simulink model "S4_LP_SCR_bypass_2018b"  (R2018b)
settings: Solver=VariableStepAuto  StartTime=0.0  StopTime=20000  RelTol=1e-3
undefined symbols (not defined in the file or in its folder): sigbuilder_block
libraries: fl_lib x70, sh_lib x49, nesl_utility x29
(part 2 of 2)

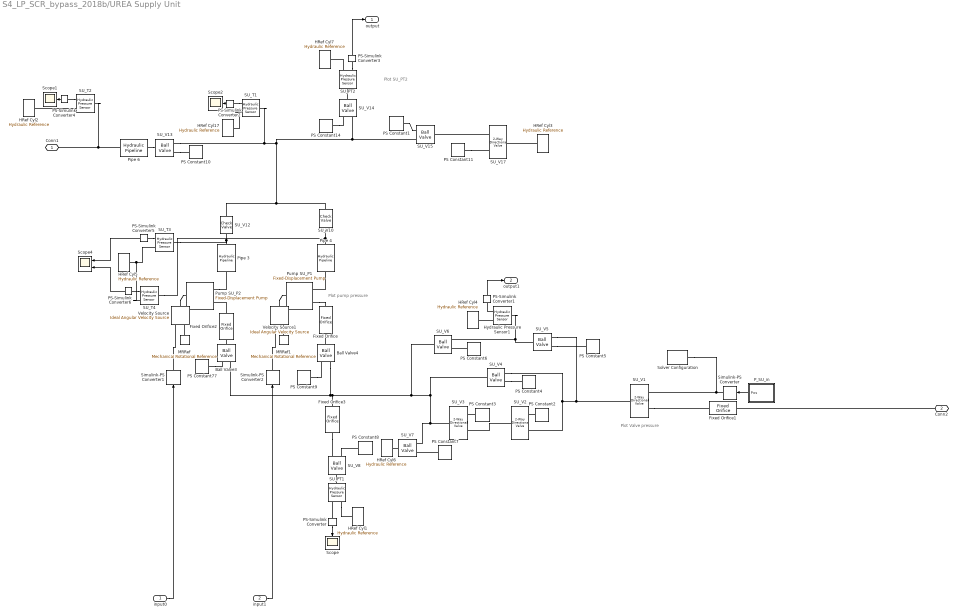
== system S4_LP_SCR_bypass_2018b/UREA Supply Unit ==
  note: Plot Valve pressure
  note: Plot pump pressure
  note: Plot SU_PT2
  input0 : Inport
  input1 : Inport  Port=2
  Ball Valve3 : sh_lib/Valves/Flow Control Valves/Ball Valve  valve_seat_spec=1  cone_ang=120 deg  d_ball=0.01 m  d_orif=5e-3 m  x_0=0 m  C_d=0.65  A_leak=1e-20 m^2  lam_spec=1  B_lam=0.999  Re_cr=10  flow_rate_specify=off  flow_rate_priority=None  flow_rate=1e-3 m^3/s  flow_rate_nominal_specify=off  flow_rate_nominal_unit=m^3/s  flow_rate_nominal_value=1  pressure_drop_specify=off  pressure_drop_priority=None  pressure_drop=0 Pa  pressure_drop_nominal_specify=off  pressure_drop_nominal_unit=Pa  pressure_drop_nominal_value=1
      settings: SourceProductBaseCode=SH  InternalSimscapePortConfiguration="{\"Bottom\":[],\"Left\":[{\"id\":\"S\",\"label\":\"S\",\"type\":\"input\"},{\"id\":\"A\",\"label\":\"A\",\"type\":\"foundation.hydraulic.hydraulic\"}],\"Right\":[{\"id\":\"B\",\"label\":\"B\",\"type\":\"foundation.hydraulic.hydraulic\"}],\"Top\":[]}"
  Ball Valve4 : sh_lib/Valves/Flow Control Valves/Ball Valve  valve_seat_spec=1  cone_ang=120 deg  d_ball=0.01 m  d_orif=5e-3 m  x_0=0 m  C_d=0.65  A_leak=1e-20 m^2  lam_spec=1  B_lam=0.999  Re_cr=10  flow_rate_specify=off  flow_rate_priority=None  flow_rate=1e-3 m^3/s  flow_rate_nominal_specify=off  flow_rate_nominal_unit=m^3/s  flow_rate_nominal_value=1  pressure_drop_specify=off  pressure_drop_priority=None  pressure_drop=0 Pa  pressure_drop_nominal_specify=off  pressure_drop_nominal_unit=Pa  pressure_drop_nominal_value=1
      settings: SourceProductBaseCode=SH  InternalSimscapePortConfiguration="{\"Bottom\":[],\"Left\":[{\"id\":\"S\",\"label\":\"S\",\"type\":\"input\"},{\"id\":\"A\",\"label\":\"A\",\"type\":\"foundation.hydraulic.hydraulic\"}],\"Right\":[{\"id\":\"B\",\"label\":\"B\",\"type\":\"foundation.hydraulic.hydraulic\"}],\"Top\":[]}"
  Fixed Orifice{,1..3} (4 alike) : sh_lib/Orifices/Fixed Orifice  area=1e-4 m^2  C_d=0.7  lam_spec=1  B_lam=0.999  Re_cr=12  q_specify=off  q_priority=None  q=1e-3 m^3/s  q_nominal_specify=off  q_nominal_unit=m^3/s  q_nominal_value=1  p_specify=off  p_priority=None  p=0 Pa  p_nominal_specify=off  p_nominal_unit=Pa  p_nominal_value=1
      settings: SourceProductBaseCode=SH  InternalSimscapePortConfiguration="{\"Bottom\":[],\"Left\":[{\"id\":\"A\",\"label\":\"A\",\"type\":\"foundation.hydraulic.hydraulic\"}],\"Right\":[{\"id\":\"B\",\"label\":\"B\",\"type\":\"foundation.hydraulic.hydraulic\"}],\"Top\":[]}"
  HRef Cyl{1..7,17} (8 alike) : fl_lib/Hydraulic/Hydraulic Elements/Hydraulic Reference  Tag=Factory Generic
      settings: SourceProductBaseCode=PW,SS,VE
  Hydraulic Pressure Sensor1 : fl_lib/Hydraulic/Hydraulic Sensors/Hydraulic Pressure Sensor
      settings: SourceProductBaseCode=PW,SS,VE
  MRRef : fl_lib/Mechanical/Rotational Elements/Mechanical Rotational Reference  Tag=Factory Generic
      settings: SourceProductBaseCode=PW,SS,VE
  MRRef1 : fl_lib/Mechanical/Rotational Elements/Mechanical Rotational Reference  Tag=Factory Generic
      settings: SourceProductBaseCode=PW,SS,VE
  PS Constant{1..3,6,11,14} (6 alike) : fl_lib/Physical Signals/Sources/PS Constant  constant=1
      settings: SourceProductBaseCode=PW,SS,VE
  PS Constant10 : fl_lib/Physical Signals/Sources/PS Constant  constant=1 m
      settings: SourceProductBaseCode=PW,SS,VE
  PS Constant4 : fl_lib/Physical Signals/Sources/PS Constant  constant=0 m
      settings: SourceProductBaseCode=PW,SS,VE
  PS Constant5 : fl_lib/Physical Signals/Sources/PS Constant  constant=1 m
      settings: SourceProductBaseCode=PW,SS,VE
  PS Constant7 : fl_lib/Physical Signals/Sources/PS Constant  constant=0 m
      settings: SourceProductBaseCode=PW,SS,VE
  PS Constant77 : fl_lib/Physical Signals/Sources/PS Constant  constant=0.01 m
      settings: SourceProductBaseCode=PW,SS,VE
  PS Constant8 : fl_lib/Physical Signals/Sources/PS Constant  constant=1 m
      settings: SourceProductBaseCode=PW,SS,VE
  PS Constant9 : fl_lib/Physical Signals/Sources/PS Constant  constant=0.01 m
      settings: SourceProductBaseCode=PW,SS,VE
  PS-Simulink Converter{,1..6} (7 alike) : nesl_utility/PS-Simulink Converter  PhysicalDomain=network_engine_domain  SubClassName=ps_output  LeftPortType=input  RightPortType=output  PseudoPeriodic=off  Frequencies=[]  VectorFormat=inherit  Unit=inherit  AffineConversion=off
      settings: SourceProductBaseCode=SS,PW,VE
  P_SU_in : Subsystem  Tag=STV Subsys  LoadFcn=sigbuilder_block('load');  StartFcn=sigbuilder_block('start');  StopFcn=sigbuilder_block('stop');  ClipboardFcn=sigbuilder_block('clipboard');  mask(Sigbuilder block){tuvar=[0:10]}
      mask help: Sigbuilder GUI
      mask init:
      | if ~strcmp(get_param(bdroot(gcbh),'SimulationStatus'),'stopped') tuvar = sigbuilder_block('maskInit'); end
      settings: CopyFcn=sigbuilder_block('copy');  DeleteFcn=sigbuilder_block('delete');  ModelCloseFcn=sigbuilder_block('modelClose');  PreSaveFcn=sigbuilder_block('preSave');  PauseFcn=sigbuilder_block('pause')  ContinueFcn=sigbuilder_block('continue')  NameChangeFcn=sigbuilder_block('namechange');  OpenFcn=sigbuilder_block('open',[0 0 787.5 524.25 ]);  CloseFcn=sigbuilder_block('close');
      mask Display: plot(0, 0, 100, 100,[2, 2, 32, 32, 2], [68, 8, 8, 68, 68],[32, 2], [38, 38], [32, 19, 2],[53, 60, 44], [32, 17, 17, 2],[16, 16, 31, 31]);txt = getActiveGroup(gcbh);text(2, 100, txt,'verticalAlignment', 'top');
  Pipe 3 : sh_lib/Pipelines/Hydraulic Pipeline  Tag=Factory Generic  cs_type=1  d_in=0.016 m  area=1e-04 m^2  D_h=0.0112 m  s_factor=64  length=5 m  length_ad=1 m  roughness=1.5e-05 m  Re_lam=2e+03  Re_turb=4e+03  wall_type=1  pr_r_coef=2e-10 m/Pa  time_const=0.008 s  k_sh=1.4  initial_pressure=0 Pa
      settings: SourceProductBaseCode=SH  InternalSimscapePortConfiguration="{\"Bottom\":[],\"Left\":[{\"id\":\"A\",\"label\":\"A\",\"type\":\"foundation.hydraulic.hydraulic\"}],\"Right\":[{\"id\":\"B\",\"label\":\"B\",\"type\":\"foundation.hydraulic.hydraulic\"}],\"Top\":[]}"
  Pipe 4 : sh_lib/Pipelines/Hydraulic Pipeline  Tag=Factory Generic  cs_type=1  d_in=0.015 m  area=1e-04 m^2  D_h=0.0112 m  s_factor=64  length=1 m  length_ad=1 m  roughness=1.5e-06 m  Re_lam=2e+03  Re_turb=4e+03  wall_type=1  pr_r_coef=2e-10 m/Pa  time_const=0.008 s  k_sh=1.4  initial_pressure=0 Pa
      settings: SourceProductBaseCode=SH  InternalSimscapePortConfiguration="{\"Bottom\":[],\"Left\":[{\"id\":\"A\",\"label\":\"A\",\"type\":\"foundation.hydraulic.hydraulic\"}],\"Right\":[{\"id\":\"B\",\"label\":\"B\",\"type\":\"foundation.hydraulic.hydraulic\"}],\"Top\":[]}"
  Pipe 6 : sh_lib/Pipelines/Hydraulic Pipeline  Tag=Factory Generic  cs_type=1  d_in=0.016 m  area=1e-04 m^2  D_h=0.0112 m  s_factor=1  length=5 m  length_ad=1 m  roughness=1.5e-05 m  Re_lam=2e+03  Re_turb=4e+03  wall_type=1  pr_r_coef=2e-10 m/Pa  time_const=0.008 s  k_sh=1.4  initial_pressure=0 Pa
      settings: SourceProductBaseCode=SH  LogSimulationData=on  InternalSimscapePortConfiguration="{\"Bottom\":[],\"Left\":[{\"id\":\"A\",\"label\":\"A\",\"type\":\"foundation.hydraulic.hydraulic\"}],\"Right\":[{\"id\":\"B\",\"label\":\"B\",\"type\":\"foundation.hydraulic.hydraulic\"}],\"Top\":[]}"
  Pump SU_P1 : sh_lib/Pumps and Motors/Fixed-Displacement Pump  D=3.2 cm^3/rev  loss_spec=1  w_nominal=200 rad/s  pr_nominal=5e7 Pa  visc_nominal=18 cSt  dens_nominal=1032.38 kg/m^3  efficiency_vol=0.92  no_load_torque=0.05 N*m  torque_pressure_coeff=0.6e-6 N*m/Pa  p_diff_eff_TLU=[100000, 1000000, 2000000] Pa  omega_eff_TLU=[25, 50, 100, 200, 300, 400] rad/s  vol_eff_TLU=[.816, .908, .954, .977, .981, .984; .325, .663, .831, .916, .925, .946; .137, .568, .78, .892, .893, .91]  mech_eff_TLU=[.996, .996, .996, .996, .996, .996; .988, .989, .989, .989, .989, .99; .981, .981, .982, .982, .983, .984]  p_diff_loss_TLU=[100000, 1000000, 2000000] Pa  omega_loss_TLU=[25, 50, 100, 200, 300, 400] rad/s  vol_loss_TLU=[.023, .023, .023, .023, .0285, .032; .0844, .0842, .0845, .084, .1125, .108; .1079, .108, .11, .108, .1605, .18] * 1e-3 m^3/s  mech_loss_TLU=[.002, .002, .002, .002, .002, .002; .0607, .0556, .0556, .0556, .0556, .0505; .1937, .1937, .1833, .1833, .1729, .1626] N*m  pressure_threshold=1e5 Pa  omega_threshold=10 rad/s  quadrant_check=0  pressure_check=0  min_valid_pressure=0 Pa  vol_eff_min=1e-3  vol_eff_max=1  mech_eff_min=1e-3  mech_eff_max=1
      settings: SourceProductBaseCode=SH  LogSimulationData=on  InternalSimscapePortConfiguration="{\"Bottom\":[],\"Left\":[{\"id\":\"S\",\"label\":\"S\",\"type\":\"foundation.mechanical.rotational.rotational\"}],\"Right\":[{\"id\":\"P\",\"label\":\"P\",\"type\":\"foundation.hydraulic.hydraulic\"},{\"id\":\"T\",\"label\":\"T\",\"type\":\"foundation.hydraulic.hydraulic\"}],\"Top\":[]}"
  Pump SU_P2 : sh_lib/Pumps and Motors/Fixed-Displacement Pump  D=3.2 cm^3/rev  loss_spec=1  w_nominal=188 rad/s  pr_nominal=100e5 Pa  visc_nominal=18 cSt  dens_nominal=900 kg/m^3  efficiency_vol=0.92  no_load_torque=0.05 N*m  torque_pressure_coeff=0.6e-6 N*m/Pa  p_diff_eff_TLU=[100000, 1000000, 2000000] Pa  omega_eff_TLU=[25, 50, 100, 200, 300, 400] rad/s  vol_eff_TLU=[.816, .908, .954, .977, .981, .984; .325, .663, .831, .916, .925, .946; .137, .568, .78, .892, .893, .91]  mech_eff_TLU=[.996, .996, .996, .996, .996, .996; .988, .989, .989, .989, .989, .99; .981, .981, .982, .982, .983, .984]  p_diff_loss_TLU=[100000, 1000000, 2000000] Pa  omega_loss_TLU=[25, 50, 100, 200, 300, 400] rad/s  vol_loss_TLU=[.023, .023, .023, .023, .0285, .032; .0844, .0842, .0845, .084, .1125, .108; .1079, .108, .11, .108, .1605, .18] * 1e-3 m^3/s  mech_loss_TLU=[.002, .002, .002, .002, .002, .002; .0607, .0556, .0556, .0556, .0556, .0505; .1937, .1937, .1833, .1833, .1729, .1626] N*m  pressure_threshold=1e5 Pa  omega_threshold=10 rad/s  quadrant_check=0  pressure_check=0  min_valid_pressure=0 Pa  vol_eff_min=1e-3  vol_eff_max=1  mech_eff_min=1e-3  mech_eff_max=1
      settings: SourceProductBaseCode=SH  InternalSimscapePortConfiguration="{\"Bottom\":[],\"Left\":[{\"id\":\"S\",\"label\":\"S\",\"type\":\"foundation.mechanical.rotational.rotational\"}],\"Right\":[{\"id\":\"P\",\"label\":\"P\",\"type\":\"foundation.hydraulic.hydraulic\"},{\"id\":\"T\",\"label\":\"T\",\"type\":\"foundation.hydraulic.hydraulic\"}],\"Top\":[]}"
  SU_PT1 : fl_lib/Hydraulic/Hydraulic Sensors/Hydraulic Pressure Sensor
      settings: SourceProductBaseCode=PW,SS,VE
  SU_PT2 : fl_lib/Hydraulic/Hydraulic Sensors/Hydraulic Pressure Sensor
      settings: SourceProductBaseCode=PW,SS,VE
  SU_T{1..4} (4 alike) : fl_lib/Hydraulic/Hydraulic Sensors/Hydraulic Pressure Sensor
      settings: SourceProductBaseCode=PW,SS,VE
  SU_V{1..3,17} (4 alike) : sh_lib/Valves/Directional Valves/2-Way Directional Valve  Tag=Factory Generic  mdl_type=1  area_max=2.2e-4 m^2  opening_max=0.01 m  opening_tab="[  -0.002 0 0.005 0.015 ] m"  area_tab="[  1e-12 4e-12 1e-05 1.02e-05 ] m^2"  pressure_tab="[  -5e+06 -2e+06 2e+06 5e+06 ] Pa"  flow_rate_tab="[  -1e-12 -6e-14 6e+12 1e+11 ; -8e-08 -4e-08 4e+06 8e+06 ; -0.0025 -0.00103 0.001 0.0024 ; -0.00258 -0.001032 0.00106 0.00247 ; ] m^3/s"  interp_method=1  extrap_method=1  C_d=0.7  x_0=8.0e-4 m  A_leak=1e-12 m^2  lam_spec=1  B_lam=0.999  Re_cr=12
      settings: SourceProductBaseCode=SH  LogSimulationData=on  InternalSimscapePortConfiguration="{\"Bottom\":[],\"Left\":[{\"id\":\"S\",\"label\":\"S\",\"type\":\"input\"},{\"id\":\"A\",\"label\":\"A\",\"type\":\"foundation.hydraulic.hydraulic\"}],\"Right\":[{\"id\":\"B\",\"label\":\"B\",\"type\":\"foundation.hydraulic.hydraulic\"}],\"Top\":[]}"
  SU_V10 : sh_lib/Valves/Directional Valves/Check Valve  area_max=1e-4 m^2  pres_crack=0.3e5 Pa  pres_max=1.2e5 Pa  C_d=0.7  A_leak=1e-12 m^2  lam_spec=1  B_lam=0.999  Re_cr=12  dynamic=0  tau=0.1 s  area_init=1e-12 m^2
      settings: SourceProductBaseCode=SH  InternalSimscapePortConfiguration="{\"Bottom\":[],\"Left\":[{\"id\":\"A\",\"label\":\"A\",\"type\":\"foundation.hydraulic.hydraulic\"}],\"Right\":[{\"id\":\"B\",\"label\":\"B\",\"type\":\"foundation.hydraulic.hydraulic\"}],\"Top\":[]}"
  SU_V12 : sh_lib/Valves/Directional Valves/Check Valve  area_max=1e-4 m^2  pres_crack=0.3e5 Pa  pres_max=1.2e5 Pa  C_d=0.7  A_leak=1e-12 m^2  lam_spec=1  B_lam=0.999  Re_cr=12  dynamic=0  tau=0.1 s  area_init=1e-12 m^2
      settings: SourceProductBaseCode=SH  InternalSimscapePortConfiguration="{\"Bottom\":[],\"Left\":[{\"id\":\"A\",\"label\":\"A\",\"type\":\"foundation.hydraulic.hydraulic\"}],\"Right\":[{\"id\":\"B\",\"label\":\"B\",\"type\":\"foundation.hydraulic.hydraulic\"}],\"Top\":[]}"
  SU_V13 : sh_lib/Valves/Flow Control Valves/Ball Valve  valve_seat_spec=1  cone_ang=120 deg  d_ball=0.01 m  d_orif=5e-3 m  x_0=0 m  C_d=8  A_leak=1e-20 m^2  lam_spec=1  B_lam=0.999  Re_cr=10  flow_rate_specify=off  flow_rate_priority=None  flow_rate=1e-3 m^3/s  flow_rate_nominal_specify=off  flow_rate_nominal_unit=m^3/s  flow_rate_nominal_value=1  pressure_drop_specify=off  pressure_drop_priority=None  pressure_drop=0 Pa  pressure_drop_nominal_specify=off  pressure_drop_nominal_unit=Pa  pressure_drop_nominal_value=1
      settings: SourceProductBaseCode=SH  InternalSimscapePortConfiguration="{\"Bottom\":[],\"Left\":[{\"id\":\"S\",\"label\":\"S\",\"type\":\"input\"},{\"id\":\"A\",\"label\":\"A\",\"type\":\"foundation.hydraulic.hydraulic\"}],\"Right\":[{\"id\":\"B\",\"label\":\"B\",\"type\":\"foundation.hydraulic.hydraulic\"}],\"Top\":[]}"
  SU_V{4..8,14..15} (7 alike) : sh_lib/Valves/Flow Control Valves/Ball Valve  valve_seat_spec=1  cone_ang=120 deg  d_ball=0.01 m  d_orif=5e-3 m  x_0=0 m  C_d=0.65  A_leak=1e-20 m^2  lam_spec=1  B_lam=0.999  Re_cr=10  flow_rate_specify=off  flow_rate_priority=None  flow_rate=1e-3 m^3/s  flow_rate_nominal_specify=off  flow_rate_nominal_unit=m^3/s  flow_rate_nominal_value=1  pressure_drop_specify=off  pressure_drop_priority=None  pressure_drop=0 Pa  pressure_drop_nominal_specify=off  pressure_drop_nominal_unit=Pa  pressure_drop_nominal_value=1
      settings: SourceProductBaseCode=SH  InternalSimscapePortConfiguration="{\"Bottom\":[],\"Left\":[{\"id\":\"S\",\"label\":\"S\",\"type\":\"input\"},{\"id\":\"A\",\"label\":\"A\",\"type\":\"foundation.hydraulic.hydraulic\"}],\"Right\":[{\"id\":\"B\",\"label\":\"B\",\"type\":\"foundation.hydraulic.hydraulic\"}],\"Top\":[]}"
  Scope : Scope
  Scope1 : Scope
  Scope2 : Scope
  Scope4 : Scope  NumInputPorts=2
  Simulink-PS Converter : nesl_utility/Simulink-PS Converter  PhysicalDomain=network_engine_domain  SubClassName=ps_input  LeftPortType=input  RightPortType=output  PseudoPeriodic=off  Frequencies=[]  NoiseDistribution=none  NoiseParameters=[]  Unit=m  AffineConversion=off  FilteringAndDerivatives=zero  SimscapeFilterOrder=1  InputFilterTimeConstant=.001  UdotUserProvided=0
      settings: SourceProductBaseCode=SS,PW,VE
  Simulink-PS Converter1 : nesl_utility/Simulink-PS Converter  PhysicalDomain=network_engine_domain  SubClassName=ps_input  LeftPortType=input  RightPortType=output  PseudoPeriodic=off  Frequencies=[]  NoiseDistribution=none  NoiseParameters=[]  Unit=1  AffineConversion=off  FilteringAndDerivatives=zero  SimscapeFilterOrder=1  InputFilterTimeConstant=.001  UdotUserProvided=0
      settings: SourceProductBaseCode=SS,PW,VE
  Simulink-PS Converter2 : nesl_utility/Simulink-PS Converter  PhysicalDomain=network_engine_domain  SubClassName=ps_input  LeftPortType=input  RightPortType=output  PseudoPeriodic=off  Frequencies=[]  NoiseDistribution=none  NoiseParameters=[]  Unit=1  AffineConversion=off  FilteringAndDerivatives=zero  SimscapeFilterOrder=1  InputFilterTimeConstant=.001  UdotUserProvided=0
      settings: SourceProductBaseCode=SS,PW,VE
  Solver Configuration : nesl_utility/Solver Configuration  PhysicalDomain=network_engine_domain  SubClassName=solver  LeftPortType=input  RightPortType=generic  Tones=[]  Harmonics=[]  SimulateNoise=off  Profile=off  UseLocalSampling=off  EnableSwitchedLinearOptims=on  FrequencyDomain=off  UseCCode=off  RelTol=0.001  AbsTol=1e-06  MinStep=1e-09  ToWorkspace=off  RevertToSquareIcSolve=off  NumHomotopyIterations=100  PhasorMode=off  PhasorModeNumHarmonics=1  IndexReductionMethod=DerivativeReplacement  DoDC=off  ResidualTolerance=1e-9  UseLocalSolver=off  LocalSolverChoice=NE_BACKWARD_EULER_ADVANCER  LocalSolverSampleTime=.001  DoFixedCost=off  MaxNonlinIter=3  MaxModeIter=2  ComputeImpulses=off  ImpulseIterations=2  LinearAlgebra=auto  LinearAlgebraNumThread=0  EquationFormulation=NE_TIME_EF  DelaysMemoryBudget=1024  AutomaticFiltering=on  FilteringTimeConstant=0.001  PartitionStorageMethod=AS_NEEDED  PartitionMemoryBudget=1024  PartitionMethod=FAST
      settings: SourceProductBaseCode=SS,PW,VE
  Velocity Source : fl_lib/Mechanical/Mechanical Sources/Ideal Angular Velocity Source  Tag=Factory Generic
      settings: SourceProductBaseCode=PW,SS,VE
  Velocity Source1 : fl_lib/Mechanical/Mechanical Sources/Ideal Angular Velocity Source  Tag=Factory Generic
      settings: SourceProductBaseCode=PW,SS,VE
  Conn1 : PMIOPort  Side=Right
  Conn2 : PMIOPort  Port=2  Side=Left
  output : Outport
  output1 : Outport  Port=2
  wires:
  P_SU_in/1(Pos) -> Simulink-PS Converter/1
  input1/1 -> Simulink-PS Converter2/1
  PS-Simulink Converter/1 -> Scope/1
  input0/1 -> Simulink-PS Converter1/1
  PS-Simulink Converter2/1 -> Scope2/1
  PS-Simulink Converter3/1 -> output/1
  PS-Simulink Converter1/1 -> output1/1
  PS-Simulink Converter4/1 -> Scope1/1
  PS-Simulink Converter5/1 -> Scope4/1
  PS-Simulink Converter6/1 -> Scope4/2
  connections:
  SU_V5/LConn1 -- PS Constant5/RConn1
  Fixed Orifice3/RConn1 -- SU_V8/LConn2
  SU_V10/RConn1 -- SU_V12/RConn1 -- SU_V15/LConn2 -- SU_V14/LConn2 -- SU_V13/LConn2 -- SU_T1/LConn1
  Simulink-PS Converter/RConn1 -- SU_V1/LConn1 -- Solver Configuration/RConn1
  Pump SU_P1/RConn2 -- Fixed Orifice/RConn1
  SU_V6/LConn2 -- SU_V5/RConn1 -- Hydraulic Pressure Sensor1/LConn1
  PS-Simulink Converter/LConn1 -- SU_PT1/RConn2
  Hydraulic Pressure Sensor1/RConn1 -- HRef Cyl4/LConn1
  Ball Valve4/RConn1 -- Fixed Orifice/LConn1
  PS Constant2/RConn1 -- SU_V2/LConn1
  SU_V4/LConn1 -- PS Constant4/RConn1
  Ball Valve4/LConn2 -- Fixed Orifice3/LConn1 -- SU_V4/RConn1 -- SU_V7/LConn2 -- SU_V3/RConn1 -- SU_V6/RConn1 -- Ball Valve3/LConn2
  PS Constant77/RConn1 -- Ball Valve3/LConn1
  PS Constant9/RConn1 -- Ball Valve4/LConn1
  SU_V13/LConn1 -- PS Constant10/RConn1
  MRRef/LConn1 -- Velocity Source/RConn2
  PS Constant14/RConn1 -- SU_V14/LConn1
  Simulink-PS Converter2/RConn1 -- Velocity Source1/RConn1
  SU_PT2/RConn1 -- HRef Cyl7/LConn1
  PS Constant6/RConn1 -- SU_V6/LConn1
  PS Constant11/RConn1 -- SU_V17/LConn1
  Hydraulic Pressure Sensor1/RConn2 -- PS-Simulink Converter1/LConn1
  Simulink-PS Converter1/RConn1 -- Velocity Source/RConn1
  SU_PT1/RConn1 -- HRef Cyl1/LConn1
  PS Constant1/RConn1 -- SU_V15/LConn1
  Fixed Orifice2/RConn1 -- Pump SU_P2/RConn2
  SU_V2/LConn2 -- SU_V4/LConn2 -- SU_V1/RConn1 -- SU_V5/LConn2
  Velocity Source/LConn1 -- Pump SU_P2/LConn1
  SU_V1/LConn2 -- Fixed Orifice1/RConn1
  Fixed Orifice2/LConn1 -- Ball Valve3/RConn1
  SU_V17/LConn2 -- SU_V15/RConn1
  SU_V12/LConn1 -- SU_T3/LConn1 -- Pipe 3/RConn1
  Velocity Source1/LConn1 -- Pump SU_P1/LConn1
  PS-Simulink Converter3/LConn1 -- SU_PT2/RConn2
  SU_PT2/LConn1 -- SU_V14/RConn1
  Pump SU_P2/RConn1 -- Pipe 3/LConn1
  SU_V10/LConn1 -- SU_T4/LConn1 -- Pipe 4/RConn1
  PS Constant8/RConn1 -- SU_V8/LConn1
  PS Constant3/RConn1 -- SU_V3/LConn1
  SU_V8/RConn1 -- SU_PT1/LConn1
  Pipe 4/LConn1 -- Pump SU_P1/RConn1
  HRef Cyl3/LConn1 -- SU_V17/RConn1
  SU_V7/RConn1 -- HRef Cyl6/LConn1
  PS Constant7/RConn1 -- SU_V7/LConn1
  MRRef1/LConn1 -- Velocity Source1/RConn2
  SU_V2/RConn1 -- SU_V3/LConn2
  Conn1/RConn1 -- SU_T2/LConn1 -- Pipe 6/RConn1
  PS-Simulink Converter2/LConn1 -- SU_T1/RConn2
  SU_T1/RConn1 -- HRef Cyl17/LConn1
  Conn2/RConn1 -- Fixed Orifice1/LConn1
  SU_T2/RConn1 -- HRef Cyl2/LConn1
  PS-Simulink Converter4/LConn1 -- SU_T2/RConn2
  Pipe 6/LConn1 -- SU_V13/RConn1
  PS-Simulink Converter5/LConn1 -- SU_T3/RConn2
  SU_T3/RConn1 -- SU_T4/RConn1 -- HRef Cyl5/LConn1
  PS-Simulink Converter6/LConn1 -- SU_T4/RConn2

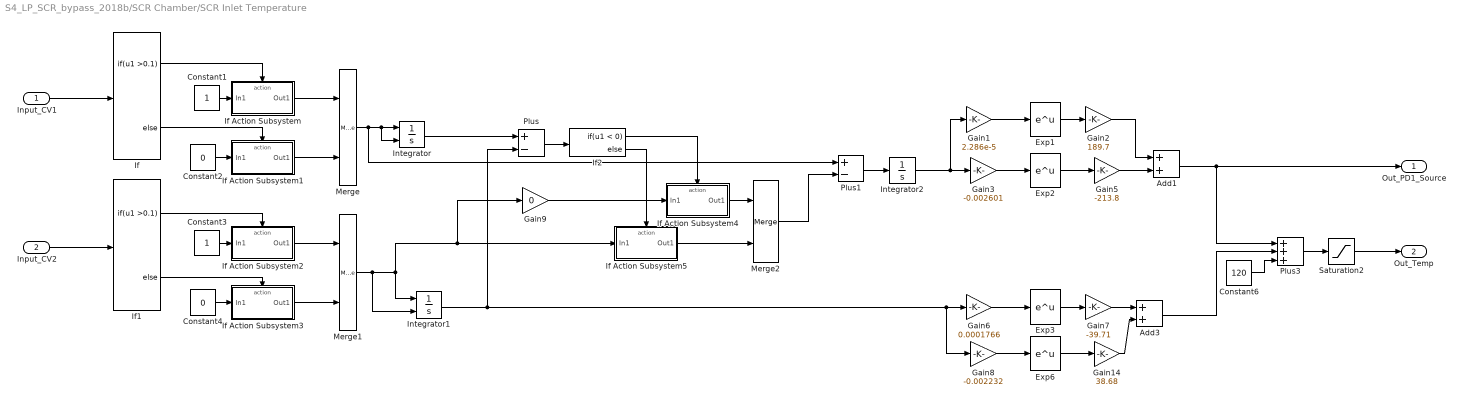
== system S4_LP_SCR_bypass_2018b/SCR Chamber/SCR Inlet Temperature ==
  Input_CV1 : Inport
  Input_CV2 : Inport  Port=2
  Add1 : Sum
  Add3 : Sum
  Constant1 : Constant
  Constant2 : Constant  Value=0
  Constant3 : Constant
  Constant4 : Constant  Value=0
  Constant6 : Constant  Value=120
  Exp{1..3,6} (4 alike) : Math  SaturateOnIntegerOverflow=on
  Gain1 : Gain  Gain=2.286e-5
  Gain14 : Gain  Gain=38.68
  Gain2 : Gain  Gain=189.7
  Gain3 : Gain  Gain=-0.002601
  Gain5 : Gain  Gain=-213.8
  Gain6 : Gain  Gain=0.0001766
  Gain7 : Gain  Gain=-39.71
  Gain8 : Gain  Gain=-0.002232
  Gain9 : Gain  Gain=0
  If : If  IfExpression=u1 >0.1  ZeroCross=off
  If Action Subsystem : Subsystem  TreatAsAtomicUnit=on
  If Action Subsystem1 : Subsystem  TreatAsAtomicUnit=on
  If Action Subsystem2 : Subsystem  TreatAsAtomicUnit=on
  If Action Subsystem3 : Subsystem  TreatAsAtomicUnit=on
  If Action Subsystem4 : Subsystem  TreatAsAtomicUnit=on
  If Action Subsystem5 : Subsystem  TreatAsAtomicUnit=on
  If1 : If  IfExpression=u1 >0.1  ZeroCross=off
  If2 : If  IfExpression=u1 < 0
  Integrator : Integrator  ExternalReset=falling
  Integrator1 : Integrator  ExternalReset=falling
  Integrator2 : Integrator
  Merge : Merge
  Merge1 : Merge
  Merge2 : Merge
  Plus : Sum  Inputs=+-
  Plus1 : Sum  Inputs=+-
  Plus3 : Sum  Inputs=+++
  Saturation2 : Saturate  UpperLimit=360  LowerLimit=120
  Out_PD1_Source : Outport
  Out_Temp : Outport  Port=2
  wires:
  If Action Subsystem3/1(Out1) -> Merge1/2
  If/1 -> If Action Subsystem/Action
  Exp3/1 -> Gain7/1
  Gain6/1 -> Exp3/1
  Constant6/1 -> Plus3/3
  If1/1 -> If Action Subsystem2/Action
  Add3/1 -> Plus3/2
  If2/2 -> If Action Subsystem5/Action
  Merge1/1 -> Integrator1/2, Integrator1/1, If Action Subsystem5/1(In1), Gain9/1
  Gain7/1 -> Add3/1
  Gain5/1 -> Add1/2
  Gain8/1 -> Exp6/1
  Constant2/1 -> If Action Subsystem1/1(In1)
  If/2 -> If Action Subsystem1/Action
  Merge/1 -> Integrator/1, Integrator/2, Plus1/1
  Gain14/1 -> Add3/2
  Add1/1 -> Out_PD1_Source/1, Plus3/1
  Plus/1 -> If2/1
  Plus3/1 -> Saturation2/1
  If Action Subsystem1/1(Out1) -> Merge/2
  Exp6/1 -> Gain14/1
  Constant1/1 -> If Action Subsystem/1(In1)
  If1/2 -> If Action Subsystem3/Action
  If Action Subsystem/1(Out1) -> Merge/1
  Merge2/1 -> Plus1/2
  Plus1/1 -> Integrator2/1
  Gain9/1 -> If Action Subsystem4/1(In1)
  If Action Subsystem2/1(Out1) -> Merge1/1
  Input_CV1/1 -> If/1
  Integrator2/1 -> Gain1/1, Gain3/1
  Saturation2/1 -> Out_Temp/1
  If2/1 -> If Action Subsystem4/Action
  Gain2/1 -> Add1/1
  Integrator1/1 -> Gain8/1, Gain6/1, Plus/2
  Constant4/1 -> If Action Subsystem3/1(In1)
  Exp1/1 -> Gain2/1
  If Action Subsystem4/1(Out1) -> Merge2/1
  Integrator/1 -> Plus/1
  Constant3/1 -> If Action Subsystem2/1(In1)
  If Action Subsystem5/1(Out1) -> Merge2/2
  Gain1/1 -> Exp1/1
  Gain3/1 -> Exp2/1
  Exp2/1 -> Gain5/1
  Input_CV2/1 -> If1/1

== system S4_LP_SCR_bypass_2018b/UREA Supply Unit/P_SU_in ==
  Demux : Demux  Tag=STV Demux  Outputs=1
      settings: DisplayOption=none
  FromWs : FromWorkspace  Tag=STV FromWs  VariableName=tuvar
      SigBuilderData=|
      | common.afterFinalStr = 'Extrapolate'
      | common.sampleTime = 0
      | dataSet.timeRange = [0 10]
      | dataSet.name = 'Group 1'
      | sbobj.Groups.Name = 'Group 1'
      | sbobj.Groups.Signals.Name = 'Pos'
      | sbobj.Groups.Signals.XData = [0 10]
      | sbobj.Groups.Signals.YData = [1 1]
  Pos : Outport  Tag=STV Outport  VectorParamsAs1DForOutWhenUnconnected=off
  wires:
  Demux/1 -> Pos/1
  FromWs/1 -> Demux/1

== system S4_LP_SCR_bypass_2018b/SCR Chamber/SCR Inlet Temperature/If Action Subsystem ==
  In1 : Inport
  Action Port : ActionPort
  Out1 : Outport
  wires:
  In1/1 -> Out1/1

== system S4_LP_SCR_bypass_2018b/SCR Chamber/SCR Inlet Temperature/If Action Subsystem1 ==
  In1 : Inport
  Action Port : ActionPort
  Out1 : Outport
  wires:
  In1/1 -> Out1/1

== system S4_LP_SCR_bypass_2018b/SCR Chamber/SCR Inlet Temperature/If Action Subsystem2 ==
  In1 : Inport
  Action Port : ActionPort
  Out1 : Outport
  wires:
  In1/1 -> Out1/1

== system S4_LP_SCR_bypass_2018b/SCR Chamber/SCR Inlet Temperature/If Action Subsystem3 ==
  In1 : Inport
  Action Port : ActionPort
  Out1 : Outport
  wires:
  In1/1 -> Out1/1

== system S4_LP_SCR_bypass_2018b/SCR Chamber/SCR Inlet Temperature/If Action Subsystem4 ==
  In1 : Inport
  Action Port : ActionPort
  Out1 : Outport
  wires:
  In1/1 -> Out1/1

== system S4_LP_SCR_bypass_2018b/SCR Chamber/SCR Inlet Temperature/If Action Subsystem5 ==
  In1 : Inport
  Action Port : ActionPort
  Out1 : Outport
  wires:
  In1/1 -> Out1/1
